simulink model "simul4knn_explicite"  (R2023b)
settings: Solver=ode4  StartTime=0.0  StopTime=240  FixedStep=0.004  RelTol=1e-3
InitFcn:
  | start4_infer_knn
StopFcn:
  | stop4_infer
values from neighbouring files (symbols this model uses):
  biais_acc = 0.003    [params4.m]    (also in start4.m)
undefined symbols (not defined in the file or in its folder): a_dlpf, b_dlpf
libraries: simulink x1
settings Model: Creator=xavie  LastModifiedBy=xavie
settings DataIOCC: ReturnWorkspaceOutputs=off

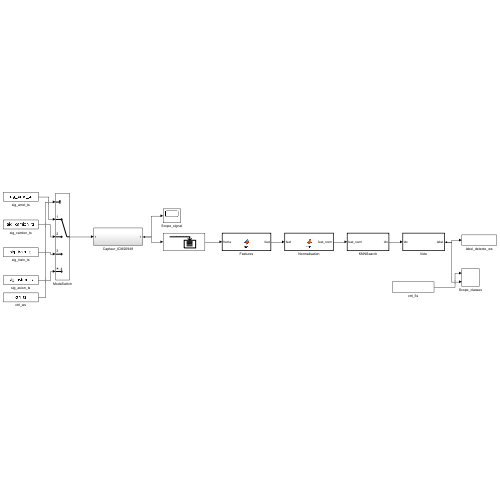
[thumbnail: Simulink's stored preview of the top-level diagram]
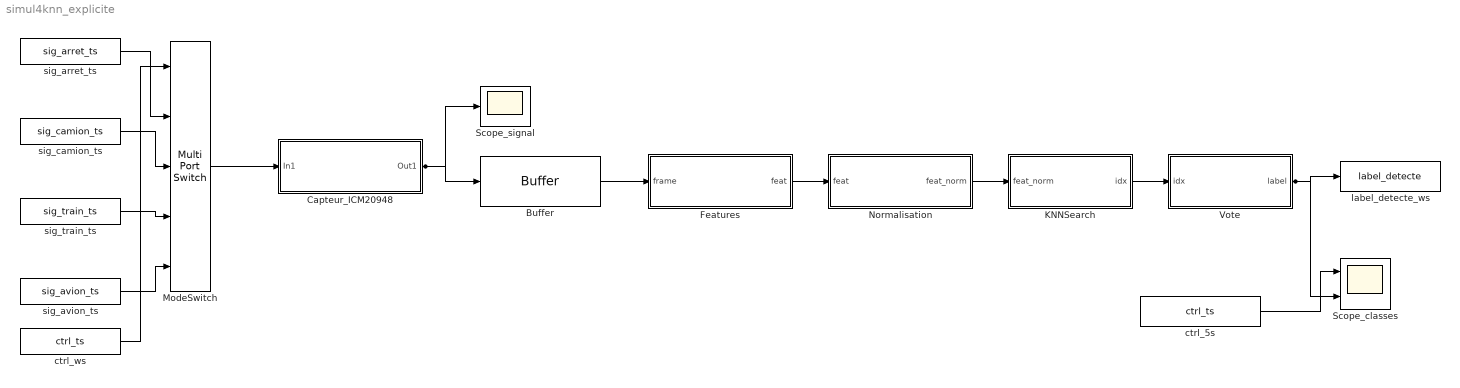
== system simul4knn_explicite ==
  Buffer : Buffer  N=2500  OverlapPercent=50
  Capteur_ICM20948 : Subsystem
  Features : MATLAB Function  TreatAsAtomicUnit=on
  KNNSearch : MATLAB Function  TreatAsAtomicUnit=on
  ModeSwitch : MultiPortSwitch  Inputs=4  SaturateOnIntegerOverflow=off  InputSameDT=off
  Normalisation : MATLAB Function  TreatAsAtomicUnit=on
  Scope_classes : Scope  NumInputPorts=2
  Scope_signal : Scope
  Vote : MATLAB Function  TreatAsAtomicUnit=on
  ctrl_5s : FromWorkspace  VariableName=ctrl_ts  SampleTime=5  Interpolate=off  OutputAfterFinalValue=Holding final value
  ctrl_ws : FromWorkspace  VariableName=ctrl_ts  SampleTime=0.004  Interpolate=off  OutputAfterFinalValue=Holding final value
  label_detecte_ws : ToWorkspace  VariableName=label_detecte  SampleTime=-1
  sig_arret_ts : FromWorkspace  VariableName=sig_arret_ts  SampleTime=0.004  Interpolate=off  OutputAfterFinalValue=Holding final value
  sig_avion_ts : FromWorkspace  VariableName=sig_avion_ts  SampleTime=0.004  Interpolate=off  OutputAfterFinalValue=Holding final value
  sig_camion_ts : FromWorkspace  VariableName=sig_camion_ts  SampleTime=0.004  Interpolate=off  OutputAfterFinalValue=Holding final value
  sig_train_ts : FromWorkspace  VariableName=sig_train_ts  SampleTime=0.004  Interpolate=off  OutputAfterFinalValue=Holding final value
  wires:
  ctrl_ws/1 -> ModeSwitch/1
  sig_arret_ts/1 -> ModeSwitch/2
  sig_camion_ts/1 -> ModeSwitch/3
  sig_train_ts/1 -> ModeSwitch/4
  sig_avion_ts/1 -> ModeSwitch/5
  ModeSwitch/1 -> Capteur_ICM20948/1(In1)
  Capteur_ICM20948/1(Out1) -> Scope_signal/1, Buffer/1
  Buffer/1 -> Features/1(frame)
  Features/1(feat) -> Normalisation/1(feat)
  Normalisation/1(feat_norm) -> KNNSearch/1(feat_norm)
  KNNSearch/1(idx) -> Vote/1(idx)
  Vote/1(label) -> label_detecte_ws/1, Scope_classes/2
  ctrl_5s/1 -> Scope_classes/1

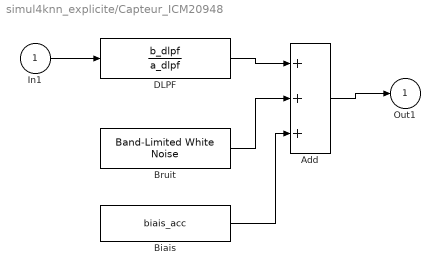
== system simul4knn_explicite/Capteur_ICM20948 ==
  In1 : Inport
  Add : Sum  Inputs=+++
  Biais : Constant  Value=biais_acc
  Bruit : simulink/Sources/Band-Limited White Noise  Cov=7.2e-09  Ts=0.004  seed=9999
  DLPF : DiscreteTransferFcn  Numerator=b_dlpf  Denominator=a_dlpf  SampleTime=0.004
  Out1 : Outport
  wires:
  In1/1 -> DLPF/1
  DLPF/1 -> Add/1
  Bruit/1 -> Add/2
  Biais/1 -> Add/3
  Add/1 -> Out1/1

== matlab function simul4knn_explicite/Features ==
  data: frame input; feat output
function feat = features_fn(frame)
%FEATURES_FN  Extraction de 6 primitives spectrales sur une fenetre de 2500 pts
%  Entree : frame  vecteur 2500x1 (issu du bloc Buffer DSP, cadence T_hop = 5 s)
%  Sortie : feat   vecteur 1x6 [RMS, crete, f_centroid, E_basse, E_milieu, E_haute]
%
%  Le bloc Buffer DSP ne sort qu'une fenetre complete par appel :
%  le calcul est donc systematique (pas de garde sur les zeros).
%#codegen
fs_loc = 250;
N_loc  = 2500;

x = frame;

rms_val  = sqrt(mean(x.^2));
crete    = max(abs(x)) / (rms_val + 1e-12);

X_fft    = abs(fft(x)).^2 / (N_loc * fs_loc);
X_one    = X_fft(1:N_loc/2+1);
X_one(2:end-1) = 2 * X_one(2:end-1);
f_v      = (0:N_loc/2)' * fs_loc / N_loc;
df_loc   = fs_loc / N_loc;
E_tot    = sum(X_one) * df_loc + 1e-12;

f_c      = sum(f_v .* X_one) * df_loc / E_tot;
E_basse  = sum(X_one(f_v >= 1  & f_v <  5 )) * df_loc / E_tot;
E_milieu = sum(X_one(f_v >= 5  & f_v < 50 )) * df_loc / E_tot;
E_haute  = sum(X_one(f_v >= 50 & f_v < 125)) * df_loc / E_tot;

feat = [rms_val, crete, f_c, E_basse, E_milieu, E_haute];
end

== matlab function simul4knn_explicite/KNNSearch ==
  data: feat_norm input; idx output
function idx = knn_search_fn(feat_norm)
%KNN_SEARCH_FN  Recherche des k=3 plus proches voisins dans X_train normalise
%  Entree : feat_norm  vecteur 1x6 (normalise par normalisation_fn)
%  Sortie : idx        vecteur 1x3 (indices dans X_train, base 1)
%#codegen
coder.extrinsic('knn_search_wrapper');

idx = zeros(1, 3);
idx = knn_search_wrapper(feat_norm);
end

== matlab function simul4knn_explicite/Vote ==
  data: idx input; label output
function label = vote_fn(idx)
%VOTE_FN  Vote majoritaire sur les labels des k plus proches voisins
%  Entree : idx   vecteur 1x3 (indices dans y_train, retournes par knn_search_fn)
%  Sortie : label scalaire  1=Arret  2=Camion  3=Train  4=Avion
%#codegen
coder.extrinsic('vote_wrapper');

label = double(0);
label = vote_wrapper(idx);
end

== matlab function simul4knn_explicite/Normalisation ==
  data: feat input; feat_norm output
function feat_norm = normalisation_fn(feat)
%NORMALISATION_FN  Normalise les features (z-score) avec les parametres du k-NN entraine
%  Entree : feat      vecteur 1x6 (issu de features_fn)
%  Sortie : feat_norm vecteur 1x6 normalise
%  mu_train et sigma_train lus depuis le workspace (mis en place par start4_infer_knn.m)
%#codegen
coder.extrinsic('evalin');

persistent mu sig
if isempty(mu)
    mu  = zeros(1, 6);
    sig = ones(1, 6);
    mu  = evalin('base', 'mu_train');
    sig = evalin('base', 'sigma_train');
end

feat_norm = (feat - mu) ./ sig;
end
